simulink model "floribot_accu_watchdog"  (R2013a)
settings: Solver=FixedStepDiscrete  SolverMode=SingleTasking  StartTime=0.0  StopTime=inf  FixedStep=0.1  RelTol=1e-3  SampleTimeConstraint=STIndependent
settings Model: Creator=Torsten  LastModifiedBy=Torsten
settings OptimizationCC: OptimizeModelRefInitCode=on  LifeSpan=Inf
settings HardwareCC: ProdLargestAtomicInteger=Long  ProdLargestAtomicFloat=Double  ProdIntDivRoundTo=Zero  ProdEndianess=LittleEndian  ProdHWDeviceType=Generic->32-bit x86 compatible
settings RTWCC: SystemTargetFile=ert.tlc  GenCodeOnly=on  GenerateMakefile=off  TemplateMakefile=ert_default_tmf  Description=Embedded Coder  ProcessScript=ert_make_rtw_hook  TargetLang=C++
settings CodeAppCC: IgnoreCustomStorageClasses=off
settings ERTTargetCC: InlinedParameterPlacement=Hierarchical  ERTCustomFileTemplate=example_file_process.tlc

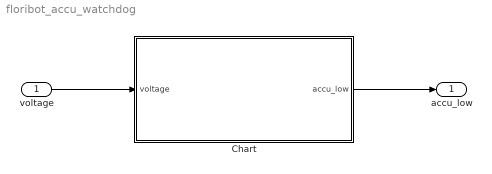
== system floribot_accu_watchdog ==
  voltage : Inport
  Chart : Stateflow chart  TreatAsAtomicUnit=on
  accu_low : Outport
  wires:
  voltage/1 -> Chart/1(voltage)
  Chart/1(accu_low) -> accu_low/1

== stateflow chart floribot_accu_watchdog/Chart ==
  state Accu_ok
    accu_low = false;
  state Accu_low
    accu_low = true;
  (default) -> Accu_ok
  Accu_ok -> Accu_low : [voltage < 10]
  Accu_low -> Accu_ok : [voltage > 10]
  data: voltage input double; accu_low output boolean
